simulink model "Prac02_3"  (R2015a)
settings: Solver=ode45  StartTime=0.0  StopTime=8  RelTol=1e-3
libraries: dsparch4 x1, dspsigops x1
settings Model: Creator=Josemi  LastModifiedBy=Josemi

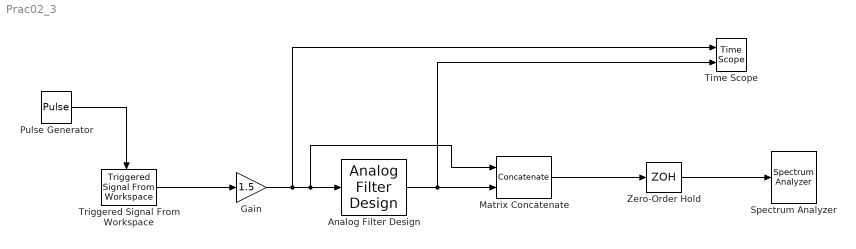
== system Prac02_3 ==
  Analog Filter Design : dsparch4/Analog Filter Design  method=Chebyshev I  filttype=Lowpass  N=8  Wlo=2*pi*80  Whi=80  Rp=6  Rs=40
  Gain : Gain  Gain=1.5
  Matrix Concatenate : Concatenate  Mode=Multidimensional array  ConcatenateDimension=2
  Pulse Generator : DiscretePulseGenerator  PulseType=Time based  Amplitude=0.5  Period=1  PulseWidth=50
  Spectrum Analyzer : SpectrumAnalyzer
  Time Scope : TimeScope  DefaultConfigurationName=spbscopes.TimeScopeBlockCfg  NumInputPorts=2
  Triggered Signal From Workspace : dspsigops/Triggered Signal From Workspace  Signal=[ 1 0 1 0 0 0 1 1 1 0 1 1 0 0 0]  TriggerType=Either edge  ic=0  SamplesPerFrame=1  OutputAfterFinalValue=Setting to zero
  Zero-Order Hold : ZeroOrderHold  SampleTime=0.0025
  wires:
  Pulse Generator/1 -> Triggered Signal From Workspace/Trigger
  Triggered Signal From Workspace/1 -> Gain/1
  Gain/1 -> Time Scope/1, Matrix Concatenate/1, Analog Filter Design/1
  Analog Filter Design/1 -> Time Scope/2, Matrix Concatenate/2
  Matrix Concatenate/1 -> Zero-Order Hold/1
  Zero-Order Hold/1 -> Spectrum Analyzer/1
